simulink model "cic_strukturen1"  (Simulink 7.8)
settings: Solver=ode45  StartTime=0.0  StopTime=10.0  RelTol=1e-3
libraries: dspsigops x4
settings Model: Creator=svenhoffmann  LastModifiedBy=josef  ExtModeAutoUpdateStatusClock=off
settings OptimizationCC: InlineInvariantSignals=on  InitFltsAndDblsToZero=on
settings DebuggingCC: SaveWithParameterizedLinksMsg=none  SignalResolutionControl=TryResolveAllWithWarning  MultiTaskDSMMsg=warning  MultiTaskCondExecSysMsg=none  StrictBusMsg=None
settings RTWCC: IncludeERTFirstTime=on
settings GRTTargetCC: TargetFcnLib=ansi_tfl_tmw.mat

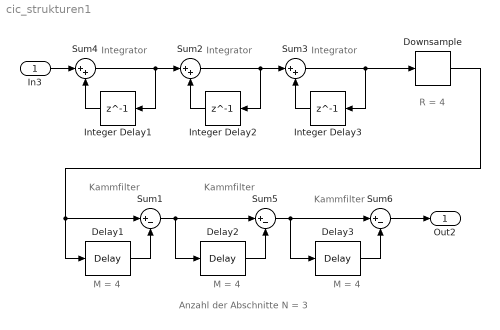
== system cic_strukturen1 ==
  note: Integrator
  note: M = 4
  note: Kammfilter
  note: R = 4
  note: Integrator
  note: Integrator
  note: M = 4
  note: M = 4
  note: Kammfilter
  note: Kammfilter
  note: Anzahl der Abschnitte N = 3
  In3 : Inport
  Delay1 : dspsigops/Delay  InputProcessing=Inherited (this choice will be removed - see release notes)  dly_unit=Samples  delay=M  ic_detail=off  dif_ic_for_ch=off  dif_ic_for_dly=off  ic=0  reset_popup=None
  Delay2 : dspsigops/Delay  InputProcessing=Inherited (this choice will be removed - see release notes)  dly_unit=Samples  delay=M  ic_detail=off  dif_ic_for_ch=off  dif_ic_for_dly=off  ic=0  reset_popup=None
  Delay3 : dspsigops/Delay  InputProcessing=Inherited (this choice will be removed - see release notes)  dly_unit=Samples  delay=M  ic_detail=off  dif_ic_for_ch=off  dif_ic_for_dly=off  ic=0  reset_popup=None
  Downsample : dspsigops/Downsample  N=4  phase=0  InputProcessing=Inherited (this choice will be removed - see release notes)  RateOptions=Enforce single-rate processing  smode=Allow multirate  fmode=Maintain input frame size  ic=0
  Integer Delay1 : Delay  DelayLength=1  InputProcessing=Inherited
  Integer Delay2 : Delay  DelayLength=1  InputProcessing=Inherited
  Integer Delay3 : Delay  DelayLength=1  InputProcessing=Inherited
  Sum1 : Sum  Inputs=|+-
  Sum2 : Sum  Inputs=|++
  Sum3 : Sum  Inputs=|++
  Sum4 : Sum  Inputs=|++
  Sum5 : Sum  Inputs=|+-
  Sum6 : Sum  Inputs=|+-
  Out2 : Outport
  wires:
  In3/1 -> Sum4/1
  Sum4/1 -> Integer Delay1/1, Sum2/1
  Integer Delay1/1 -> Sum4/2
  Delay1/1 -> Sum1/2
  Downsample/1 -> Delay1/1, Sum1/1
  Sum2/1 -> Integer Delay2/1, Sum3/1
  Integer Delay2/1 -> Sum2/2
  Sum3/1 -> Integer Delay3/1, Downsample/1
  Integer Delay3/1 -> Sum3/2
  Sum6/1 -> Out2/1
  Delay2/1 -> Sum5/2
  Sum1/1 -> Sum5/1, Delay2/1
  Delay3/1 -> Sum6/2
  Sum5/1 -> Delay3/1, Sum6/1
